simulink model "ysw11_22"  (R2014a)
settings: Solver=ode45  StartTime=0.0  StopTime=10.0  RelTol=1e-3
libraries: commdigbbndam3 x1
settings Model: Creator=ii  LastModifiedBy=ii
settings SolverCC: ZeroCrossAlgorithm=Adaptive
settings DebuggingCC: UnderspecifiedInitializationDetection=Classic

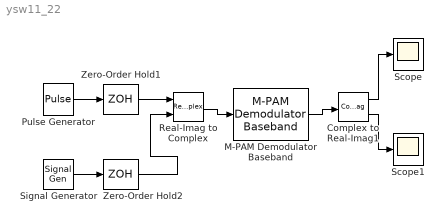
== system ysw11_22 ==
  Complex to Real-Imag1 : ComplexToRealImag
  M-PAM Demodulator Baseband : commdigbbndam3/M-PAM Demodulator Baseband  M=4  OutType=Integer  Dec=Gray  PowType=Min. distance between symbols  MinDist=2  AvgPow=1  PeakPow=1  outDtype1=Inherit via internal rule  outDtype2=Inherit via internal rule  denormFactorWordLen=16  prodOutWordLen=16  prodOutRoundingMode=Floor  prodOutOverflowMode=Wrap  sumWordLen=16
  Pulse Generator : DiscretePulseGenerator  PulseType=Time based  Amplitude=300  Period=10  PulseWidth=5
  Real-Imag to Complex : RealImagToComplex
  Scope : Scope
  Scope1 : Scope
  Signal Generator : SignalGenerator  Amplitude=100  Frequency=1000  Units=rad/sec
  Zero-Order Hold1 : ZeroOrderHold
  Zero-Order Hold2 : ZeroOrderHold
  wires:
  Complex to Real-Imag1/1 -> Scope/1
  Complex to Real-Imag1/2 -> Scope1/1
  Zero-Order Hold1/1 -> Real-Imag to Complex/1
  Pulse Generator/1 -> Zero-Order Hold1/1
  Signal Generator/1 -> Zero-Order Hold2/1
  Zero-Order Hold2/1 -> Real-Imag to Complex/2
  Real-Imag to Complex/1 -> M-PAM Demodulator Baseband/1
  M-PAM Demodulator Baseband/1 -> Complex to Real-Imag1/1
